simulink model "subModel_oneJointDynamic"  (R2018a)
settings: Solver=VariableStepAuto  StartTime=0.0  StopTime=10.0  RelTol=1e-3  EnableMultiTasking=on
model workspace: external: MATLAB File D:\Google Drive\Duongw_Folder\Thesis Master\_Model\Delta_Model_ADEPT\SIMCAPE_MULTI_BODY\ADEPT_DELTA_3AXES1\data_specMotor.m (data not in the file)
values from neighbouring files (symbols this model uses):
  G = -5    [Assem1_ADEPT_HORNET_DataFile.m]    (also in data_specMotor.m)
settings Model: Creator=ThanhUTC  LastModifiedBy=ShiningDanyang
settings OptimizationCC: LifeSpan=inf
settings DebuggingCC: SFUnexpectedBacktrackingDiag=warning  SFNoUnconditionalDefaultTransitionDiag=warning  SFExecutionAtInitializationDiag=none
settings CodeAppCC: StateflowObjectComments=on
settings GRTTargetCC: TargetLangStandard=C89/C90 (ANSI)  GeneratePreprocessorConditionals=Disable all
settings ConfigComp: CovMetricSettings=dw  CovHtmlReporting=on  CovSaveCumulativeToWorkspaceVar=on  CovSaveSingleToWorkspaceVar=on  CovExternalEMLEnable=off
settings SimscapeCC: SimscapeNormalizeSystem=off

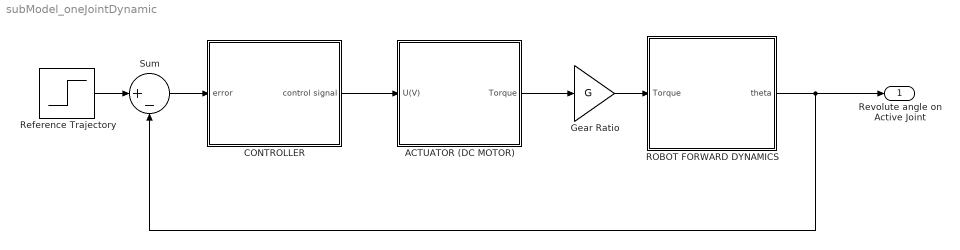
== system subModel_oneJointDynamic ==
  ACTUATOR (DC MOTOR) : Subsystem
  CONTROLLER : Subsystem
  Gear Ratio : Gain  Gain=G
  ROBOT FORWARD DYNAMICS : Subsystem
  Reference Trajectory : Step  SampleTime=0
  Sum : Sum  Inputs=|+-
  Revolute angle on Active Joint : Outport
  wires:
  ACTUATOR (DC MOTOR)/1(Torque) -> Gear Ratio/1
  ROBOT FORWARD DYNAMICS/1(theta) -> Sum/2, Revolute angle on Active Joint/1
  Gear Ratio/1 -> ROBOT FORWARD DYNAMICS/1(Torque)
  Sum/1 -> CONTROLLER/1(error)
  CONTROLLER/1(control signal) -> ACTUATOR (DC MOTOR)/1(U(V))
  Reference Trajectory/1 -> Sum/1

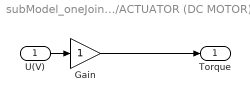
== system subModel_oneJointDynamic/ACTUATOR (DC MOTOR) ==
  U(V) : Inport
  Gain : Gain
  Torque : Outport
  wires:
  U(V)/1 -> Gain/1
  Gain/1 -> Torque/1

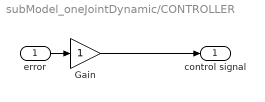
== system subModel_oneJointDynamic/CONTROLLER ==
  error : Inport
  Gain : Gain
  control signal : Outport
  wires:
  Gain/1 -> control signal/1
  error/1 -> Gain/1

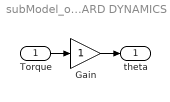
== system subModel_oneJointDynamic/ROBOT FORWARD DYNAMICS ==
  Torque : Inport
  Gain : Gain
  theta : Outport
  wires:
  Gain/1 -> theta/1
  Torque/1 -> Gain/1
